simulink model "SS4"  (R2020a)
settings: Solver=VariableStepAuto  StartTime=0.0  StopTime=10.0  RelTol=1e-3
settings Model: Creator=Asus  LastModifiedBy=Asus

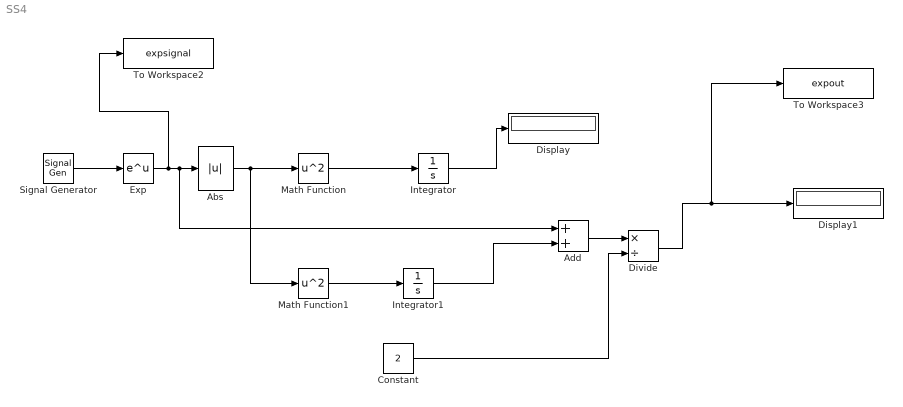
== system SS4 ==
  Abs : Abs
  Add : Sum
  Constant : Constant  Value=2
  Display : Display
  Display1 : Display
  Divide : Product  Inputs=*/
  Exp : Math  SaturateOnIntegerOverflow=on
  Integrator : Integrator  LimitOutput=on
  Integrator1 : Integrator  LimitOutput=on
  Math Function : Math  Operator=square  SaturateOnIntegerOverflow=on
  Math Function1 : Math  Operator=square  SaturateOnIntegerOverflow=on
  Signal Generator : SignalGenerator  Units=rad/sec
  To Workspace2 : ToWorkspace  VariableName=expsignal  SaveFormat=Timeseries  SampleTime=-1
  To Workspace3 : ToWorkspace  VariableName=expout  SaveFormat=Timeseries  SampleTime=-1
  wires:
  Abs/1 -> Math Function1/1, Math Function/1
  Integrator1/1 -> Add/2
  Math Function/1 -> Integrator/1
  Math Function1/1 -> Integrator1/1
  Constant/1 -> Divide/2
  Integrator/1 -> Display/1
  Signal Generator/1 -> Exp/1
  Exp/1 -> To Workspace2/1, Add/1, Abs/1
  Divide/1 -> To Workspace3/1, Display1/1
  Add/1 -> Divide/1
